simulink library "AircraftSixDOFModel"  (R2024a)
settings: Solver=VariableStepAuto  StartTime=0.0  StopTime=10.0  RelTol=1e-3
undefined symbols (not defined in the file): InertiaTensor
libraries: Aerodynamics x1, Atmosphere x1, Equations_of_Motion x1, Propulsion x1
settings Model: Creator=mahariansyah  LastModifiedBy=mahariansyah

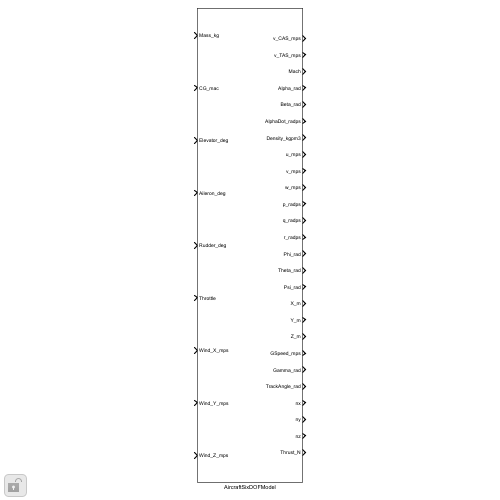
[thumbnail: Simulink's stored preview of the top-level diagram]
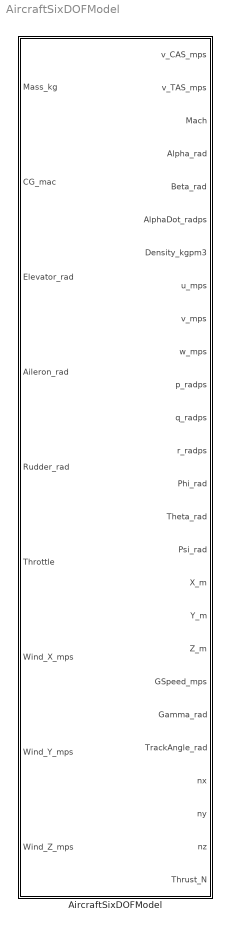
== system AircraftSixDOFModel ==
  AircraftSixDOFModel : Subsystem

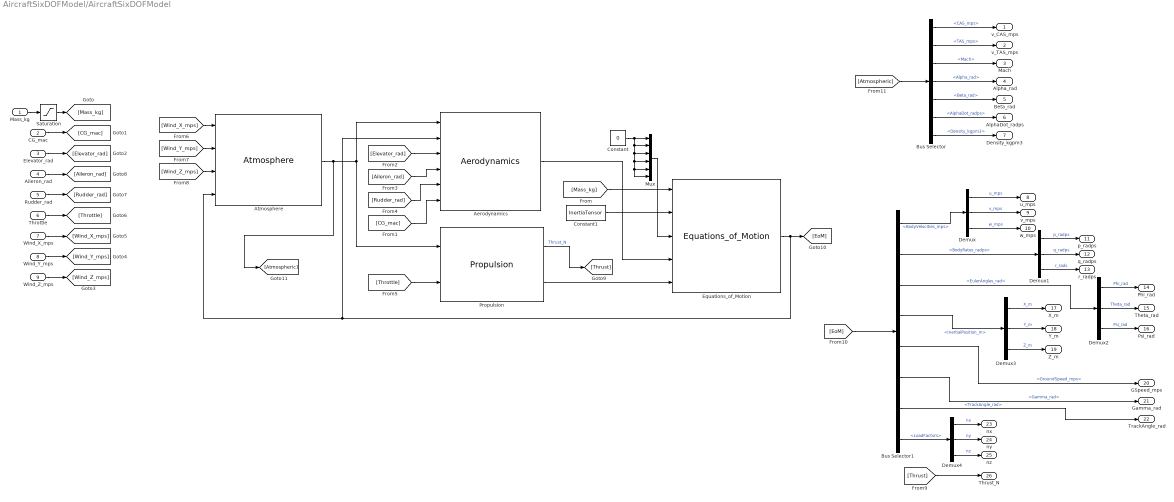
== system AircraftSixDOFModel/AircraftSixDOFModel ==
  Mass_kg : Inport
  CG_mac : Inport  Port=2
  Elevator_rad : Inport  Port=3
  Aileron_rad : Inport  Port=4
  Rudder_rad : Inport  Port=5
  Throttle : Inport  Port=6
  Wind_X_mps : Inport  Port=7
  Wind_Y_mps : Inport  Port=8
  Wind_Z_mps : Inport  Port=9
  Aerodynamics : Aerodynamics/Aerodynamics  SystemSampleTime=-1  VariantActivationTime=update diagram  AllowFlexibleInterface=on  Latency=0  AutoFrameSizeCalculation=off
  Atmosphere : Atmosphere/Atmosphere  SystemSampleTime=-1  VariantActivationTime=update diagram  AllowFlexibleInterface=on  Latency=0  AutoFrameSizeCalculation=off
  Bus Selector : BusSelector  OutputSignals=CAS_mps,TAS_mps,Mach,Alpha_rad,Beta_rad,AlphaDot_radps,Density_kgpm3
  Bus Selector1 : BusSelector  OutputSignals=BodyVelocities_mps,BodyRates_radps,EulerAngles_rad,InertialPosition_m,GroundSpeed_mps,Gamma_rad,TrackAngle_rad,LoadFactors
  Constant : Constant  Value=0
  Constant1 : Constant  Value=InertiaTensor
  Demux{,1..4} (5 alike) : Demux  Outputs=3
  Equations_of_Motion : Equations_of_Motion/Equations_of_Motion  SystemSampleTime=-1  VariantActivationTime=update diagram  AllowFlexibleInterface=on  Latency=0  AutoFrameSizeCalculation=off
  Mux : Mux  Inputs=6
  Propulsion : Propulsion/Propulsion  SystemSampleTime=-1  VariantActivationTime=update diagram  AllowFlexibleInterface=on  Latency=0  AutoFrameSizeCalculation=off
  Saturation : Saturate  UpperLimit=inf  LowerLimit=0.1
  v_CAS_mps : Outport
  v_TAS_mps : Outport  Port=2
  Mach : Outport  Port=3
  Alpha_rad : Outport  Port=4
  Beta_rad : Outport  Port=5
  AlphaDot_radps : Outport  Port=6
  Density_kgpm3 : Outport  Port=7
  u_mps : Outport  Port=8
  v_mps : Outport  Port=9
  w_mps : Outport  Port=10
  p_radps : Outport  Port=11
  q_radps : Outport  Port=12
  r_radps : Outport  Port=13
  Phi_rad : Outport  Port=14
  Theta_rad : Outport  Port=15
  Psi_rad : Outport  Port=16
  X_m : Outport  Port=17
  Y_m : Outport  Port=18
  Z_m : Outport  Port=19
  GSpeed_mps : Outport  Port=20
  Gamma_rad : Outport  Port=21
  TrackAngle_rad : Outport  Port=22
  nx : Outport  Port=23
  ny : Outport  Port=24
  nz : Outport  Port=25
  Thrust_N : Outport  Port=26
  wires:
  Demux4/3 -> nz/1  "nz"
  Demux1/3 -> r_radps/1  "r_rads"
  CG_mac/1 -> [CG_mac]
  Demux2/3 -> Psi_rad/1  "Psi_rad"
  Demux/1 -> u_mps/1  "u_mps"
  Atmosphere/1 -> [Atmospheric], Aerodynamics/1, Propulsion/1
  Demux2/2 -> Theta_rad/1  "Theta_rad"
  Demux/2 -> v_mps/1  "v_mps"
  [Wind_Y_mps] -> Atmosphere/2
  Constant1/1 -> Equations_of_Motion/2
  Mux/1 -> Equations_of_Motion/3
  Constant/1 -> Mux/1, Mux/6, Mux/5, Mux/4, Mux/3, Mux/2
  [Mass_kg] -> Equations_of_Motion/1
  Equations_of_Motion/1 -> [EoM], Atmosphere/4, Aerodynamics/2
  [Elevator_rad] -> Aerodynamics/3
  Wind_X_mps/1 -> [Wind_X_mps]
  Mass_kg/1 -> Saturation/1
  Demux3/1 -> X_m/1  "X_m"
  Demux4/2 -> ny/1  "ny"
  Demux1/1 -> p_radps/1  "p_radps"
  Propulsion/2 -> Equations_of_Motion/5
  [Rudder_rad] -> Aerodynamics/5
  Demux2/1 -> Phi_rad/1  "Phi_rad"
  Aileron_rad/1 -> [Aileron_rad]
  Wind_Z_mps/1 -> [Wind_Z_mps]
  [CG_mac] -> Aerodynamics/6
  Demux4/1 -> nx/1  "nx"
  Saturation/1 -> [Mass_kg]
  [Throttle] -> Propulsion/2
  Demux3/2 -> Y_m/1  "Y_m"
  Demux3/3 -> Z_m/1  "Z_m"
  Demux/3 -> w_mps/1  "w_mps"
  Demux1/2 -> q_radps/1  "q_radps"
  Throttle/1 -> [Throttle]
  Wind_Y_mps/1 -> [Wind_Y_mps]
  [Wind_Z_mps] -> Atmosphere/3
  Aerodynamics/1 -> Equations_of_Motion/4
  Rudder_rad/1 -> [Rudder_rad]
  Elevator_rad/1 -> [Elevator_rad]
  [Wind_X_mps] -> Atmosphere/1
  [Aileron_rad] -> Aerodynamics/4
  Bus Selector/1 -> v_CAS_mps/1  "<CAS_mps>"
  Bus Selector/2 -> v_TAS_mps/1  "<TAS_mps>"
  Bus Selector/3 -> Mach/1  "<Mach>"
  Bus Selector/4 -> Alpha_rad/1  "<Alpha_rad>"
  Bus Selector/5 -> Beta_rad/1  "<Beta_rad>"
  Bus Selector/6 -> AlphaDot_radps/1  "<AlphaDot_radps>"
  Bus Selector/7 -> Density_kgpm3/1  "<Density_kgpm3>"
  Bus Selector1/1 -> Demux/1  "<BodyVelocities_mps>"
  Bus Selector1/2 -> Demux1/1  "<BodyRates_radps>"
  Bus Selector1/3 -> Demux2/1  "<EulerAngles_rad>"
  Bus Selector1/4 -> Demux3/1  "<InertialPosition_m>"
  Bus Selector1/5 -> GSpeed_mps/1  "<GroundSpeed_mps>"
  Bus Selector1/6 -> Gamma_rad/1  "<Gamma_rad>"
  Bus Selector1/7 -> TrackAngle_rad/1  "<TrackAngle_rad>"
  Bus Selector1/8 -> Demux4/1  "<LoadFactors>"
  Propulsion/1 -> [Thrust]  "Thrust_N"
  [Thrust] -> Thrust_N/1
  [EoM] -> Bus Selector1/1
  [Atmospheric] -> Bus Selector/1
